simulink model "SrvMtr"  (R2019a)
settings: Solver=VariableStepAuto  StartTime=0.0  StopTime=10.0  RelTol=1e-3
libraries: simulink x2
settings Model: Creator=chiha  LastModifiedBy=chiha

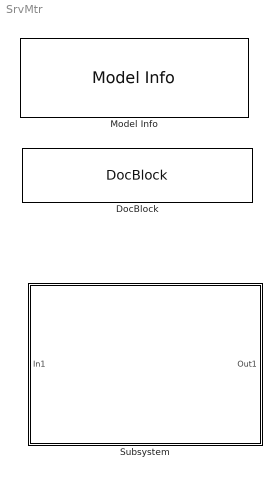
== system SrvMtr ==
  DocBlock : simulink/Model-Wide Utilities/DocBlock  DocumentType=Text
  Model Info : simulink/Model-Wide Utilities/Model Info  Frame=on  DisplayStringWithTags=|  HorizontalTextAlignment=Center  LeftAlignmentValue=0.5
      | Model Info
      | %<ModelName>
      | %<Description>
      | %<LastModificationDate>
  Subsystem : Subsystem

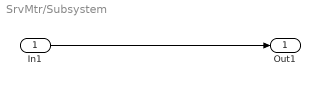
== system SrvMtr/Subsystem ==
  In1 : Inport
  Out1 : Outport
  wires:
  In1/1 -> Out1/1
